simulink model "Monitor"  (R2022b)
settings: Solver=ode1  StartTime=0.0  StopTime=0.2  FixedStep=ctrlConst.TsSwitch  MaxStep=1e-6  RelTol=1e-3  EnableMultiTasking=on
PreLoadFcn:
  | %rtwdemo_pmsmfoc_data
StartFcn:
  | %clear executionProfile
StopFcn:
  | %try
  | %  AddExecutionProfileToDataInspector();
  | %end
undefined symbols (not defined in the file or in its folder): dataIphaOfsRawMon_C, facAdc2iPhMon_C, facAdc2uDclnkMon_C, KiRslvMonPI_C, KpRslvMonPI_C, Ld, Lq, Rss, SC_pMon_P, SC_PsiMon_P, tauTrqMonLv2_C, tauUdcPT1Mon_C, trqASCThdMonLv2_C, trqCmpThdMonLv2_C, Ts_10ms, Ts_1ms, Tsw
libraries: MathLib x14, IOLib x1, simulink x1
(part 1 of 2)
settings Model: Creator=The MathWorks, Inc.  LastModifiedBy=M00039784
settings SolverCC: AlgebraicLoopSolver=TrustRegion  InsertRTBMode=Never (minimum delay)
settings DataIOCC: LimitDataPoints=on  SaveFormat=Array  SaveOutput=off  SaveTime=off
settings OptimizationCC: DefaultParameterBehavior=Inlined  UseDivisionForNetSlopeComputation=on  UseFloatMulNetSlope=on  DefaultUnderspecifiedDataType=single  InlineInvariantSignals=on  PassReuseOutputArgsAs=Individual arguments  ExpressionDepthLimit=2147483647  ZeroExternalMemoryAtStartup=off  ZeroInternalMemoryAtStartup=off  NoFixptDivByZeroProtection=on  EfficientFloat2IntCast=on  LifeSpan=1  EfficientTunableParamExpr=on
settings DebuggingCC: ReadBeforeWriteMsg=DisableAll  WriteAfterWriteMsg=DisableAll  WriteAfterReadMsg=DisableAll  AlgebraicLoopMsg=none  MultiTaskDSMMsg=none  SingleTaskRateTransMsg=error  IntegerOverflowMsg=none  ParameterPrecisionLossMsg=none  FcnCallInpInsideContextMsg=warning  BusObjectLabelMismatch=none  AssertControl=DisableAll  AllowSymbolicDim=off  StateNameClashWarn=warning  SFUnexpectedBacktrackingDiag=warning  SFNoUnconditionalDefaultTransitionDiag=warning  SFExecutionAtInitializationDiag=none  SFMachineParentedDataDiag=warning  IntegerSaturationMsg=none  UnitsInconsistencyMsg=none  ArithmeticOperatorsInVariantConditions=warning
settings HardwareCC: ProdBitPerPointer=32  ProdBitPerSizeT=32  ProdBitPerPtrDiffT=32  ProdLargestAtomicFloat=None  ProdWordSize=32  ProdHWDeviceType=Infineon->TriCore
settings ModelReferenceCC: UpdateModelReferenceTargets=IfOutOfDate  EnableRefExpFcnMdlSchedulingChecks=on  ModelReferenceNumInstancesAllowed=Single  PropagateSignalLabelsOutOfModel=off
settings SFSimCC: SFSimEcho=off  SimUseLocalCustomCode=off  MATLABDynamicMemAlloc=off  CustomCodeUndefinedFunction=UseInterfaceOnly
settings RTWCC: Description=Embedded Coder  SystemTargetFile=ert.tlc  GenCodeOnly=on  GenerateMakefile=off  TemplateMakefile=ec_target.tmf  RTWVerbose=off  RTWUseLocalCustomCode=off  PortableWordSizes=on  CodeExecutionProfiling=on  CodeProfilingSaveOptions=AllData  CodeProfilingInstrumentation=detailed
settings CodeAppCC: ForceParamTrailComments=on  IgnoreCustomStorageClasses=off  IgnoreTestpoints=on  MaxIdLength=64  SimulinkDataObjDesc=on  MATLABFcnDesc=on  CustomSymbolStrGlobalVar=monitor_rt$N$M  CustomSymbolStrType=monitor_$N$M  CustomSymbolStrFcn=$N$M$F  CustomSymbolStrFcnArg=$I$N$M  CustomSymbolStrMacro=$N$M  InsertBlockDesc=on  StateflowObjectComments=on  MATLABSourceComments=on  InternalIdentifier=Classic
settings ERTTargetCC: UtilityFuncGeneration=Shared location  MultiwordLength=2048  CombineSignalStateStructs=on  SupportAbsoluteTime=off  SupportNonFinite=off  SupportComplex=off  SupportNonInlinedSFcns=on  RemoveResetFunc=off  ParenthesesLevel=Maximum  GenerateASAP2=on  InlinedParameterPlacement=NonHierarchical  ERTCustomFileTemplate=example_file_process.tlc  EnableDataOwnership=on  ConvertIfToSwitch=off  SuppressUnreachableDefaultCases=off  MemSecPackage=Simulink  MemSecDataConstants=MemConst  MemSecDataParameters=MemConstVolatile
settings ConfigComp: CovMetricSettings=dcmtrzow  CovHTMLOptions=-aTS=1 -bRG=1 -bTC=1 -hTR=0 -nFC=0 -scm=1 -bcm=1 -xEv=0  CovSaveCumulativeToWorkspaceVar=on  CovSaveSingleToWorkspaceVar=on  CovExternalEMLEnable=off  CovSFcnEnable=off
settings SimscapeCC: SimscapeNormalizeSystem=off

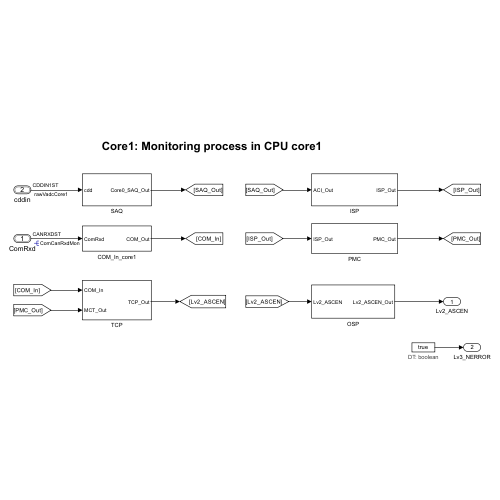
[thumbnail: Simulink's stored preview of the top-level diagram]
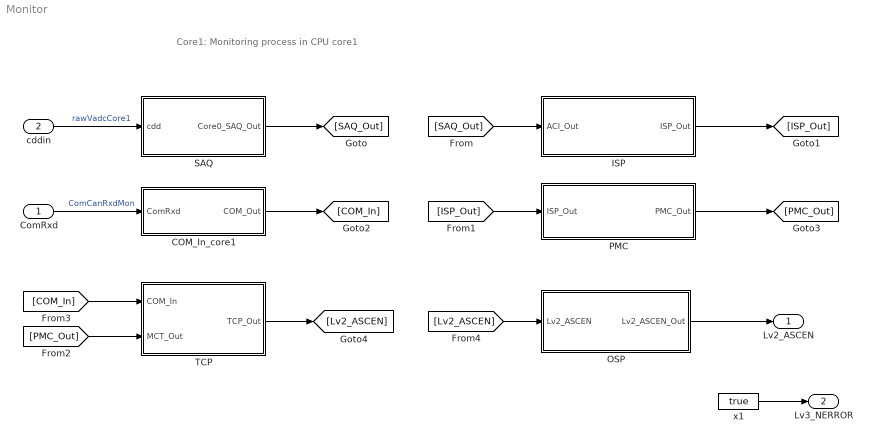
== system Monitor ==
  note: Core1: Monitoring process in CPU core1
  ComRxd : Inport  OutDataTypeStr=Bus: CANRXDST  SampleTime=Ts_10ms  BusOutputAsStruct=on
  cddin : Inport  Port=2  OutDataTypeStr=Bus: CDDIN1ST  SampleTime=Tsw  BusOutputAsStruct=on
  COM_In_core1 : Subsystem
  ISP : Subsystem
      settings: RTWSystemCode=Nonreusable function
  OSP : Subsystem
  PMC : Subsystem  SystemSampleTime=Tsw
  SAQ : Subsystem
  TCP : Subsystem  SystemSampleTime=Tsw
  x1 : Constant  Value=true  OutDataTypeStr=boolean
      settings: AttributesFormatString=DT: %<OutDataTypeStr>
  Lv2_ASCEN : Outport  VectorParamsAs1DForOutWhenUnconnected=off
  Lv3_NERROR : Outport  Port=2  VectorParamsAs1DForOutWhenUnconnected=off
  wires:
  SAQ/1(Core0_SAQ_Out) -> [SAQ_Out]
  cddin/1 -> SAQ/1(cdd)  "rawVadcCore1"
  [SAQ_Out] -> ISP/1(ACI_Out)
  ComRxd/1 -> COM_In_core1/1(ComRxd)  "ComCanRxdMon"
  COM_In_core1/1(COM_Out) -> [COM_In]
  ISP/1(ISP_Out) -> [ISP_Out]
  [ISP_Out] -> PMC/1(ISP_Out)
  PMC/1(PMC_Out) -> [PMC_Out]
  [PMC_Out] -> TCP/2(MCT_Out)
  [COM_In] -> TCP/1(COM_In)
  x1/1 -> Lv3_NERROR/1
  TCP/1(TCP_Out) -> [Lv2_ASCEN]
  [Lv2_ASCEN] -> OSP/1(Lv2_ASCEN)
  OSP/1(Lv2_ASCEN_Out) -> Lv2_ASCEN/1

== system Monitor/COM_In_core1 ==
  ComRxd : Inport  OutDataTypeStr=Bus: CANRXDST
  MSG04 : Subsystem
  Sel : BusSelector  OutputSignals=msg_MSG_04
  bus : BusCreator  Inputs=1
  COM_Out : Outport  VectorParamsAs1DForOutWhenUnconnected=off
  wires:
  ComRxd/1 -> Sel/1
  bus/1 -> COM_Out/1
  Sel/1 -> MSG04/1(MSG04)  "<msg_MSG_04>"
  MSG04/1(Com_MSG04) -> bus/1  "Com_Msg04"

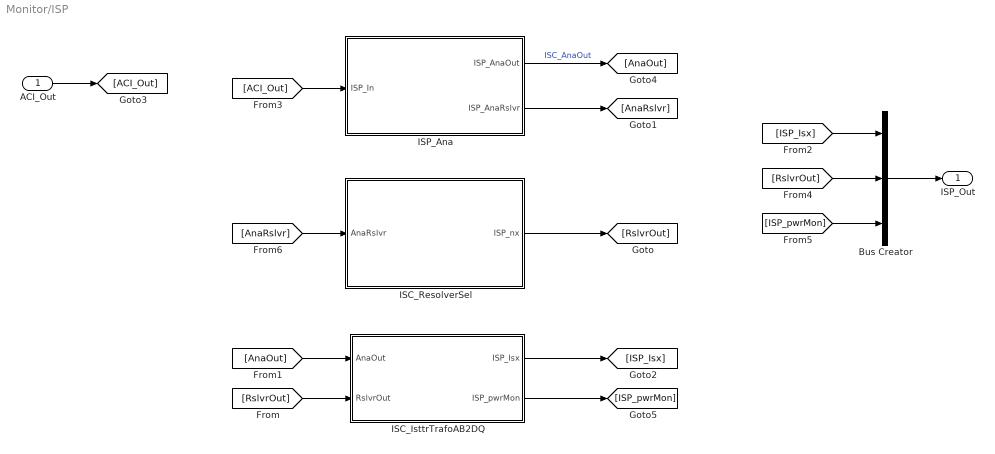
== system Monitor/ISP ==
  ACI_Out : Inport
  Bus Creator : BusCreator  Inputs=3
  ISC_IsttrTrafoAB2DQ : Subsystem
  ISC_ResolverSel : Subsystem
  ISP_Ana : Subsystem
  ISP_Out : Outport  VectorParamsAs1DForOutWhenUnconnected=off
  wires:
  ACI_Out/1 -> [ACI_Out]
  [ACI_Out] -> ISP_Ana/1(ISP_In)
  ISP_Ana/1(ISP_AnaOut) -> [AnaOut]  "ISC_AnaOut"
  [AnaOut] -> ISC_IsttrTrafoAB2DQ/1(AnaOut)
  ISP_Ana/2(ISP_AnaRslvr) -> [AnaRslvr]
  [RslvrOut] -> ISC_IsttrTrafoAB2DQ/2(RslvrOut)
  ISC_IsttrTrafoAB2DQ/1(ISP_Isx) -> [ISP_Isx]
  Bus Creator/1 -> ISP_Out/1
  [ISP_Isx] -> Bus Creator/1
  [RslvrOut] -> Bus Creator/2
  [AnaRslvr] -> ISC_ResolverSel/1(AnaRslvr)
  ISC_ResolverSel/1(ISP_nx) -> [RslvrOut]
  ISC_IsttrTrafoAB2DQ/2(ISP_pwrMon) -> [ISP_pwrMon]
  [ISP_pwrMon] -> Bus Creator/3

== system Monitor/OSP ==
  note: User is resposible to collect all the digital signals and resTolve to workspce
      | here the constant are only for reference
  Lv2_ASCEN : Inport
  SetDo7 : IOLib/SetDo  SystemSampleTime=-1
      link override Enumerated Constant: Value=EGPO.L2ASCEN
  Lv2_ASCEN_Out : Outport  VectorParamsAs1DForOutWhenUnconnected=off
  wires:
  Lv2_ASCEN/1 -> Lv2_ASCEN_Out/1

== system Monitor/PMC ==
  ISP_Out : Inport
  Bus Creator : BusCreator  Inputs=1
  Bus Selector1 : BusSelector  OutputSignals=ISP_Isx.ISP_isdMon,ISP_Isx.ISP_isqMon,ISP_nxMon.ISP_wElecMon
  PMC_PsmMdl : Subsystem
  PMC_TrqCal : Subsystem
  Terminator1 : Terminator
  Terminator2 : Terminator
  PMC_Out : Outport  VectorParamsAs1DForOutWhenUnconnected=off
  wires:
  ISP_Out/1 -> Bus Selector1/1
  Bus Selector1/1 -> PMC_PsmMdl/1(ISP_Isd)  "<ISP_isdMon>"
  Bus Selector1/2 -> PMC_PsmMdl/2(ISP_Isq)  "<ISP_isqMon>"
  Bus Selector1/3 -> PMC_PsmMdl/3(ISP_wElec)  "<ISP_wElecMon>"
  PMC_PsmMdl/1(PMC_IsdFlt1ms) -> PMC_TrqCal/1(PMC_IsdFlt1ms)
  PMC_PsmMdl/2(PMC_IsqFlt1ms) -> PMC_TrqCal/2(PMC_IsqFlt1ms)
  PMC_PsmMdl/3(PMC_PsiExc) -> PMC_TrqCal/3(PMC_psiExc)
  PMC_PsmMdl/4(PMC_LqSubLd) -> PMC_TrqCal/4(PMC_LqSubLd)
  PMC_PsmMdl/5(PMC_Ld) -> Terminator1/1
  PMC_PsmMdl/6(PMC_Rs) -> Terminator2/1
  Bus Creator/1 -> PMC_Out/1
  PMC_TrqCal/1(PMC_trqMon) -> Bus Creator/1

== system Monitor/SAQ ==
  cdd : Inport
  cddRt : Subsystem
  Core0_SAQ_Out : Outport  VectorParamsAs1DForOutWhenUnconnected=off
      settings: AttributesFormatString=Disable Action: %<OutputWhenDisabled>
  wires:
  cdd/1 -> cddRt/1(cddSt)
  cddRt/1(cddSig) -> Core0_SAQ_Out/1  "cddRt"

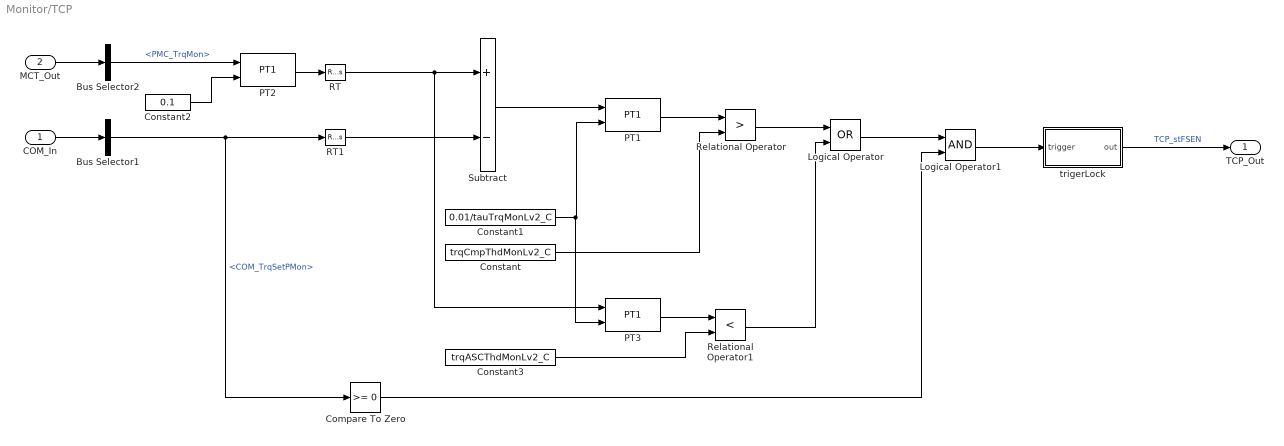
== system Monitor/TCP ==
  COM_In : Inport
  MCT_Out : Inport  Port=2
  Bus Selector1 : BusSelector  OutputSignals=Com_Msg04.COM_TrqSetPMon
  Bus Selector2 : BusSelector  OutputSignals=PMC_TrqMon
  Compare To Zero : simulink/Logic and Bit Operations/Compare To Zero  relop=>=  OutDataTypeStr=boolean
  Constant : Constant  Value=trqCmpThdMonLv2_C
  Constant1 : Constant  Value=0.01/tauTrqMonLv2_C
  Constant2 : Constant  Value=0.1
  Constant3 : Constant  Value=trqASCThdMonLv2_C
  Logical Operator : Logic  Operator=OR  AllPortsSameDT=off  OutDataTypeStr=boolean
  Logical Operator1 : Logic  AllPortsSameDT=off  OutDataTypeStr=boolean
  PT1 : MathLib/PT1
  PT2 : MathLib/PT1
  PT3 : MathLib/PT1
  RT : RateTransition  OutPortSampleTime=Ts_10ms
  RT1 : RateTransition  OutPortSampleTime=Ts_10ms
  Relational Operator : RelationalOperator  Operator=>  OutDataTypeStr=boolean  RndMeth=Simplest  InputSameDT=off
  Relational Operator1 : RelationalOperator  Operator=<  OutDataTypeStr=boolean  RndMeth=Simplest  InputSameDT=off
  Subtract : Sum  Inputs=+-
  trigerLock : MATLAB Function
  TCP_Out : Outport  VectorParamsAs1DForOutWhenUnconnected=off
  wires:
  COM_In/1 -> Bus Selector1/1
  MCT_Out/1 -> Bus Selector2/1
  Bus Selector1/1 -> Compare To Zero/1, RT1/1  "<COM_TrqSetPMon>"
  PT1/1 -> Relational Operator/1
  Constant/1 -> Relational Operator/2
  Logical Operator1/1 -> trigerLock/1(trigger)
  Subtract/1 -> PT1/1
  Constant1/1 -> PT3/2, PT1/2
  Constant2/1 -> PT2/2
  Bus Selector2/1 -> PT2/1  "<PMC_TrqMon>"
  PT2/1 -> RT/1
  RT/1 -> PT3/1, Subtract/1
  RT1/1 -> Subtract/2
  Constant3/1 -> Relational Operator1/2
  Relational Operator1/1 -> Logical Operator/2
  Logical Operator/1 -> Logical Operator1/1
  Compare To Zero/1 -> Logical Operator1/2
  trigerLock/1(out) -> TCP_Out/1  "TCP_stFSEN"
  Relational Operator/1 -> Logical Operator/1
  PT3/1 -> Relational Operator1/1

== system Monitor/COM_In_core1/MSG04 ==
  MSG04 : Inport
  Data Type Conversion : DataTypeConversion  OutDataTypeStr=Enum: ECM  SaturateOnIntegerOverflow=off  RndMeth=Floor
  Data Type Conversion1 : DataTypeConversion  OutDataTypeStr=uint16  SaturateOnIntegerOverflow=off  RndMeth=Floor
  RT{,1..3} (4 alike) : RateTransition
  Sel : BusSelector  OutputSignals=MSG04_NSetP,MSG04_TrqSetP,MSG04_UdcSetP,MSG04_stModeReq
  bus : BusCreator  Inputs=4
  Com_MSG04 : Outport  VectorParamsAs1DForOutWhenUnconnected=off
  wires:
  MSG04/1 -> Sel/1
  bus/1 -> Com_MSG04/1
  RT/1 -> bus/1  "COM_NSetPMon"
  Sel/1 -> RT/1  "<MSG04_NSetP>"
  RT1/1 -> bus/2  "COM_TrqSetPMon"
  Sel/2 -> RT1/1  "<MSG04_TrqSetP>"
  RT2/1 -> bus/3  "COM_UdcSetPMon"
  Sel/3 -> RT2/1  "<MSG04_UdcSetP>"
  RT3/1 -> bus/4  "COM_stModeReqMon"
  Sel/4 -> Data Type Conversion1/1  "<MSG04_stModeReq>"
  Data Type Conversion/1 -> RT3/1
  Data Type Conversion1/1 -> Data Type Conversion/1

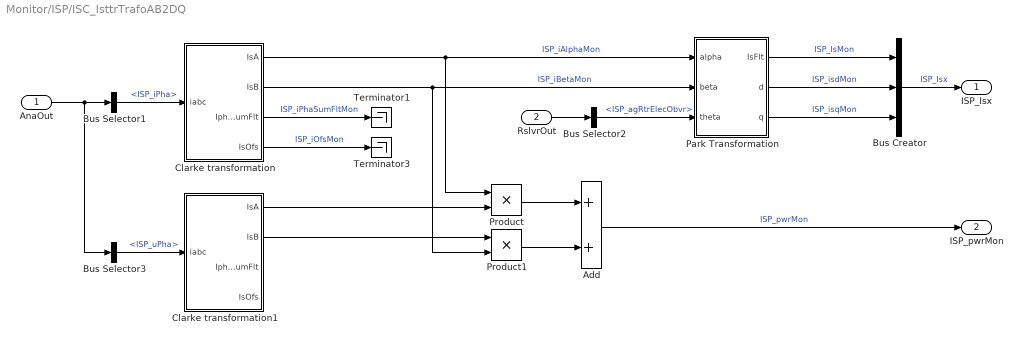
== system Monitor/ISP/ISC_IsttrTrafoAB2DQ ==
  AnaOut : Inport
  RslvrOut : Inport  Port=2
  Add : Sum
  Bus Creator : BusCreator  Inputs=3
  Bus Selector1 : BusSelector  OutputSignals=ISP_iPha
  Bus Selector2 : BusSelector  OutputSignals=ISP_agRtrElecObvr
  Bus Selector3 : BusSelector  OutputSignals=ISP_uPha
  Clarke transformation : Subsystem
  Clarke transformation1 : Subsystem
  Park Transformation : Subsystem
  Product : Product
  Product1 : Product
  Terminator1 : Terminator
  Terminator3 : Terminator
  ISP_Isx : Outport  VectorParamsAs1DForOutWhenUnconnected=off
  ISP_pwrMon : Outport  Port=2  VectorParamsAs1DForOutWhenUnconnected=off
  wires:
  Bus Creator/1 -> ISP_Isx/1  "ISP_Isx"
  Clarke transformation/4(IsOfs) -> Terminator3/1  "ISP_iOfsMon"
  AnaOut/1 -> Bus Selector3/1, Bus Selector1/1
  Park Transformation/2(d) -> Bus Creator/2  "ISP_isdMon"
  Park Transformation/3(q) -> Bus Creator/3  "ISP_isqMon"
  Clarke transformation/1(IsA) -> Product/1, Park Transformation/1(alpha)  "ISP_iAlphaMon"
  Clarke transformation/2(IsB) -> Product1/2, Park Transformation/2(beta)  "ISP_iBetaMon"
  Park Transformation/1(IsFlt) -> Bus Creator/1  "ISP_IsMon"
  Bus Selector1/1 -> Clarke transformation/1(iabc)  "<ISP_iPha>"
  Clarke transformation/3(IphaSumFlt) -> Terminator1/1  "ISP_iPhaSumFltMon"
  RslvrOut/1 -> Bus Selector2/1
  Bus Selector2/1 -> Park Transformation/3(theta)  "<ISP_agRtrElecObvr>"
  Bus Selector3/1 -> Clarke transformation1/1(iabc)  "<ISP_uPha>"
  Clarke transformation1/1(IsA) -> Product/2
  Clarke transformation1/2(IsB) -> Product1/1
  Product/1 -> Add/1
  Product1/1 -> Add/2
  Add/1 -> ISP_pwrMon/1  "ISP_pwrMon"

== system Monitor/ISP/ISC_ResolverSel ==
  note: Theta Selection
  note: if the resolver flag ture, the output angle and electric frequency are equal to the observer
      | if the resolver flag false, the output andle and electric frequency are equal to the dirct atan2 calculation.
  AnaRslvr : Inport
  Bus Creator : BusCreator  Inputs=4
  Bus Selector6 : BusSelector  OutputSignals=ISP_agRtrElecObvr,ISP_frqElecObvr
  Divide : Product  Inputs=*/
  NpMotorDivNpResolver1 : Constant  Value=SC_pMon_P  OutDataTypeStr=Inherit: Inherit via back propagation
  Saturation : Saturate  UpperLimit=18000  LowerLimit=-18000
  fac2piFrq2w : Gain  Gain=2*pi  SaturateOnIntegerOverflow=on  OutDataTypeStr=Inherit: Same as input  ParamDataTypeStr=Inherit: Same as input
  facf2n : Gain  Gain=60  SaturateOnIntegerOverflow=on  OutDataTypeStr=Inherit: Same as input  ParamDataTypeStr=Inherit: Same as input
  ISP_nx : Outport  VectorParamsAs1DForOutWhenUnconnected=off
  wires:
  AnaRslvr/1 -> Bus Selector6/1
  Bus Creator/1 -> ISP_nx/1  "ISP_nxMon"
  facf2n/1 -> Divide/1
  fac2piFrq2w/1 -> Bus Creator/3  "ISP_wElecMon"
  Bus Selector6/1 -> Bus Creator/1  "<ISP_agRtrElecObvr>"
  Bus Selector6/2 -> facf2n/1, fac2piFrq2w/1, Bus Creator/2  "<ISP_frqElecObvr>"
  Saturation/1 -> Bus Creator/4  "ISP_nMon"
  Divide/1 -> Saturation/1
  NpMotorDivNpResolver1/1 -> Divide/2

== system Monitor/ISP/ISP_Ana ==
  note: Input Signal Calculation (Analogue)
  ISP_In : Inport
  Bus Creator : BusCreator  Inputs=3
  Bus Creator1 : BusCreator  Inputs=5
  Bus Selector1 : BusSelector  OutputSignals=SAQ_SINH,SAQ_SINL,SAQ_COSH,SAQ_COSL
  Bus Selector2 : BusSelector  OutputSignals=SAQ_HVUEX
  Bus Selector3 : BusSelector  OutputSignals=SAQ_IPH1B,SAQ_IPH2B,SAQ_IPH3B  OutputAsBus=on
  Bus Selector4 : BusSelector  OutputSignals=SAQ_DUTY1,SAQ_DUTY2,SAQ_DUTY3  OutputAsBus=on
  ISP_AnaCalnIpha : Subsystem
  ISP_AnaCalnPosCalnMon : Subsystem  SystemSampleTime=Tsw
      settings: RTWSystemCode=Nonreusable function
  ISP_AnaCalnUdcLnk : Subsystem  SystemSampleTime=Tsw
  ISP_AnaCalnUpha : Subsystem
  tiPerd : Constant  Value=100  OutDataTypeStr=single
  ISP_AnaOut : Outport  VectorParamsAs1DForOutWhenUnconnected=off
  ISP_AnaRslvr : Outport  Port=2  VectorParamsAs1DForOutWhenUnconnected=off
  wires:
  ISP_In/1 -> Bus Selector3/1, Bus Selector4/1, Bus Selector1/1, Bus Selector2/1
  ISP_AnaCalnIpha/1(ISP_iPha) -> Bus Creator/2  "ISP_iPha"
  ISP_AnaCalnUdcLnk/1(ISP_uDcFltMon) -> Bus Creator/3
  Bus Creator/1 -> ISP_AnaOut/1
  Bus Selector1/1 -> ISP_AnaCalnPosCalnMon/1(sinH)  "<SAQ_SINH>"
  Bus Selector1/2 -> ISP_AnaCalnPosCalnMon/2(sinL)  "<SAQ_SINL>"
  Bus Selector1/3 -> ISP_AnaCalnPosCalnMon/3(cosH)  "<SAQ_COSH>"
  Bus Selector1/4 -> ISP_AnaCalnPosCalnMon/4(cosL)  "<SAQ_COSL>"
  tiPerd/1 -> ISP_AnaCalnPosCalnMon/5(tiPerd)
  ISP_AnaCalnPosCalnMon/3(ISP_frqElecObvr) -> Bus Creator1/3
  ISP_AnaCalnPosCalnMon/2(ISP_agRtrElecObvr) -> Bus Creator1/2
  ISP_AnaCalnPosCalnMon/4(ISP_agRtrElecAtan2) -> Bus Creator1/4
  ISP_AnaCalnPosCalnMon/1(dAngle) -> Bus Creator1/1
  ISP_AnaCalnPosCalnMon/5(ISP_frqElecCaln) -> Bus Creator1/5
  Bus Creator1/1 -> ISP_AnaRslvr/1  "ISP_RslvrOut"
  ISP_AnaCalnUpha/1(ISP_uPha) -> Bus Creator/1  "ISP_uPha"
  Bus Selector2/1 -> ISP_AnaCalnUdcLnk/1(CddHvMcu_dataDclnkRaw)  "<SAQ_HVUEX>"
  Bus Selector3/1 -> ISP_AnaCalnIpha/1(dataIPha)
  Bus Selector4/1 -> ISP_AnaCalnUpha/1(dataUPha)

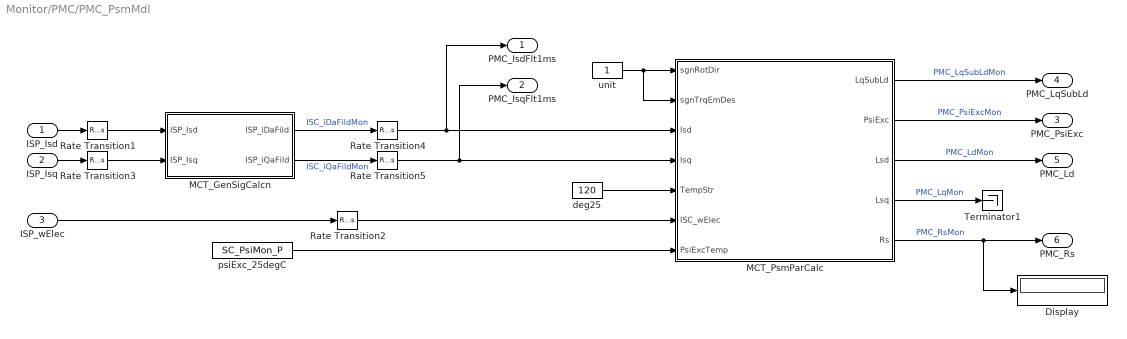
== system Monitor/PMC/PMC_PsmMdl ==
  ISP_Isd : Inport
  ISP_Isq : Inport  Port=2
  ISP_wElec : Inport  Port=3
  Display : Display
  MCT_GenSigCalcn : Subsystem
  MCT_PsmParCalc : Subsystem  TreatAsAtomicUnit=on  SystemSampleTime=Ts_1ms
  Rate Transition1 : RateTransition  OutPortSampleTime=Tsw
  Rate Transition2 : RateTransition  OutPortSampleTime=Ts_1ms
  Rate Transition3 : RateTransition  OutPortSampleTime=Tsw
  Rate Transition4 : RateTransition  OutPortSampleTime=Ts_1ms
  Rate Transition5 : RateTransition  OutPortSampleTime=Ts_1ms
  Terminator1 : Terminator
  deg25 : Constant  Value=120  OutDataTypeStr=single  SampleTime=Ts_1ms
  psiExc_25degC : Constant  Value=SC_PsiMon_P  OutDataTypeStr=single  SampleTime=Ts_1ms
  unit : Constant  OutDataTypeStr=uint8  SampleTime=Ts_1ms
  PMC_IsdFlt1ms : Outport  VectorParamsAs1DForOutWhenUnconnected=off
  PMC_IsqFlt1ms : Outport  Port=2  VectorParamsAs1DForOutWhenUnconnected=off
  PMC_PsiExc : Outport  Port=3  VectorParamsAs1DForOutWhenUnconnected=off
  PMC_LqSubLd : Outport  Port=4  VectorParamsAs1DForOutWhenUnconnected=off
  PMC_Ld : Outport  Port=5  VectorParamsAs1DForOutWhenUnconnected=off
  PMC_Rs : Outport  Port=6  VectorParamsAs1DForOutWhenUnconnected=off
  wires:
  MCT_PsmParCalc/5(Rs) -> Display/1, PMC_Rs/1  "PMC_RsMon"
  MCT_PsmParCalc/1(LqSubLd) -> PMC_LqSubLd/1  "PMC_LqSubLdMon"
  MCT_PsmParCalc/2(PsiExc) -> PMC_PsiExc/1  "PMC_PsiExcMon"
  Rate Transition5/1 -> PMC_IsqFlt1ms/1, MCT_PsmParCalc/4(Isq)
  Rate Transition3/1 -> MCT_GenSigCalcn/2(ISP_Isq)
  Rate Transition1/1 -> MCT_GenSigCalcn/1(ISP_Isd)
  MCT_GenSigCalcn/1(ISP_iDaFild) -> Rate Transition4/1  "ISC_iDaFildMon"
  ISP_Isq/1 -> Rate Transition3/1
  ISP_Isd/1 -> Rate Transition1/1
  MCT_GenSigCalcn/2(ISP_iQaFild) -> Rate Transition5/1  "ISC_iQaFildMon"
  MCT_PsmParCalc/3(Lsd) -> PMC_Ld/1  "PMC_LdMon"
  MCT_PsmParCalc/4(Lsq) -> Terminator1/1  "PMC_LqMon"
  deg25/1 -> MCT_PsmParCalc/5(TempStr)
  unit/1 -> MCT_PsmParCalc/2(sgnTrqEmDes), MCT_PsmParCalc/1(sgnRotDir)
  ISP_wElec/1 -> Rate Transition2/1
  Rate Transition2/1 -> MCT_PsmParCalc/6(ISC_wElec)
  psiExc_25degC/1 -> MCT_PsmParCalc/7(PsiExcTemp)
  Rate Transition4/1 -> PMC_IsdFlt1ms/1, MCT_PsmParCalc/3(Isd)

== system Monitor/PMC/PMC_TrqCal ==
  PMC_IsdFlt1ms : Inport
  PMC_IsqFlt1ms : Inport  Port=2
  PMC_psiExc : Inport  Port=3
  PMC_LqSubLd : Inport  Port=4
  Add : Sum  Inputs=+-
  Constant : Constant  Value=SC_pMon_P
  Constant1 : Constant  Value=3  OutDataTypeStr=single
  Product : Product
  Product1 : Product
  Product2 : Product  Inputs=3
  Product3 : Product
  PMC_trqMon : Outport  VectorParamsAs1DForOutWhenUnconnected=off
  wires:
  Product3/1 -> PMC_trqMon/1  "PMC_TrqMon"
  PMC_IsdFlt1ms/1 -> Product2/2
  PMC_IsqFlt1ms/1 -> Product2/1, Product1/2
  Constant1/1 -> Product/1
  Constant/1 -> Product/2
  PMC_psiExc/1 -> Product1/1
  PMC_LqSubLd/1 -> Product2/3
  Product1/1 -> Add/1
  Product2/1 -> Add/2
  Product/1 -> Product3/1
  Add/1 -> Product3/2

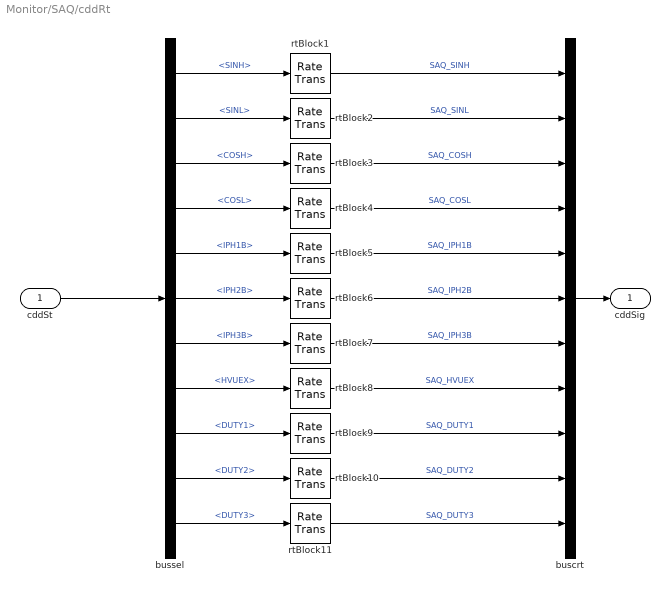
== system Monitor/SAQ/cddRt ==
  cddSt : Inport
  buscrt : BusCreator  Inputs=11
  bussel : BusSelector  OutputSignals=SINH,SINL,COSH,COSL,IPH1B,IPH2B,IPH3B,HVUEX,DUTY1,DUTY2,DUTY3
  rtBlock{1..11} (11 alike) : RateTransition  OutPortSampleTimeOpt=Inherit
  cddSig : Outport
  wires:
  cddSt/1 -> bussel/1
  buscrt/1 -> cddSig/1
  bussel/1 -> rtBlock1/1  "<SINH>"
  rtBlock1/1 -> buscrt/1  "SAQ_SINH"
  bussel/2 -> rtBlock2/1  "<SINL>"
  rtBlock2/1 -> buscrt/2  "SAQ_SINL"
  bussel/3 -> rtBlock3/1  "<COSH>"
  rtBlock3/1 -> buscrt/3  "SAQ_COSH"
  bussel/4 -> rtBlock4/1  "<COSL>"
  rtBlock4/1 -> buscrt/4  "SAQ_COSL"
  bussel/5 -> rtBlock5/1  "<IPH1B>"
  rtBlock5/1 -> buscrt/5  "SAQ_IPH1B"
  bussel/6 -> rtBlock6/1  "<IPH2B>"
  rtBlock6/1 -> buscrt/6  "SAQ_IPH2B"
  bussel/7 -> rtBlock7/1  "<IPH3B>"
  rtBlock7/1 -> buscrt/7  "SAQ_IPH3B"
  bussel/8 -> rtBlock8/1  "<HVUEX>"
  rtBlock8/1 -> buscrt/8  "SAQ_HVUEX"
  bussel/9 -> rtBlock9/1  "<DUTY1>"
  rtBlock9/1 -> buscrt/9  "SAQ_DUTY1"
  bussel/10 -> rtBlock10/1  "<DUTY2>"
  rtBlock10/1 -> buscrt/10  "SAQ_DUTY2"
  bussel/11 -> rtBlock11/1  "<DUTY3>"
  rtBlock11/1 -> buscrt/11  "SAQ_DUTY3"

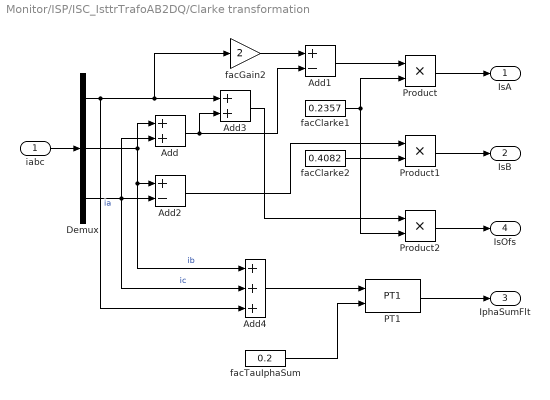
== system Monitor/ISP/ISC_IsttrTrafoAB2DQ/Clarke transformation ==
  iabc : Inport
  Add : Sum
  Add1 : Sum  Inputs=+-
  Add2 : Sum  Inputs=+-
  Add3 : Sum
  Add4 : Sum  Inputs=+++
  Demux : Demux  Outputs=3
  PT1 : MathLib/PT1
  Product : Product
  Product1 : Product  OutDataTypeStr=single
  Product2 : Product  OutDataTypeStr=single
  facClarke1 : Constant  Value=0.2357  OutDataTypeStr=single
  facClarke2 : Constant  Value=0.4082  OutDataTypeStr=single
  facGain2 : Gain  Gain=2
  facTauIphaSum : Constant  Value=0.2  OutDataTypeStr=single
  IsA : Outport  VectorParamsAs1DForOutWhenUnconnected=off
  IsB : Outport  Port=2  VectorParamsAs1DForOutWhenUnconnected=off
  IphaSumFlt : Outport  Port=3  VectorParamsAs1DForOutWhenUnconnected=off
  IsOfs : Outport  Port=4  VectorParamsAs1DForOutWhenUnconnected=off
  wires:
  Demux/1 -> Add4/3, Add3/1, facGain2/1  "ia"
  iabc/1 -> Demux/1
  Demux/3 -> Add4/2, Add2/2, Add/2  "ic"
  Demux/2 -> Add4/1, Add2/1, Add/1  "ib"
  facGain2/1 -> Add1/1
  Add/1 -> Add1/2, Add3/2
  Add1/1 -> Product/1
  Product/1 -> IsA/1
  facClarke1/1 -> Product2/2, Product/2
  Add2/1 -> Product1/1
  facClarke2/1 -> Product1/2
  Product1/1 -> IsB/1
  Add3/1 -> Product2/1
  Product2/1 -> IsOfs/1
  PT1/1 -> IphaSumFlt/1
  facTauIphaSum/1 -> PT1/2
  Add4/1 -> PT1/1

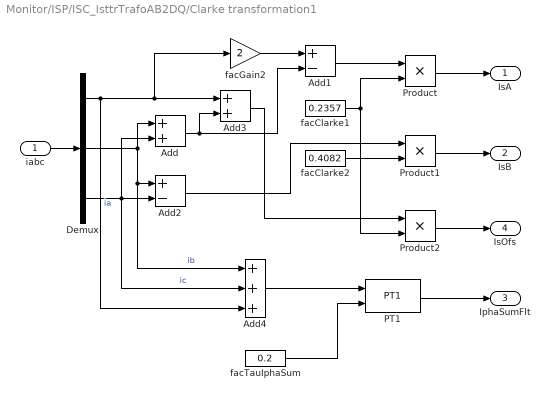
== system Monitor/ISP/ISC_IsttrTrafoAB2DQ/Clarke transformation1 ==
  iabc : Inport
  Add : Sum
  Add1 : Sum  Inputs=+-
  Add2 : Sum  Inputs=+-
  Add3 : Sum
  Add4 : Sum  Inputs=+++
  Demux : Demux  Outputs=3
  PT1 : MathLib/PT1  SystemSampleTime=-1  VariantActivationTime=update diagram  Latency=0  AutoFrameSizeCalculation=off
  Product : Product
  Product1 : Product  OutDataTypeStr=single
  Product2 : Product  OutDataTypeStr=single
  facClarke1 : Constant  Value=0.2357  OutDataTypeStr=single
  facClarke2 : Constant  Value=0.4082  OutDataTypeStr=single
  facGain2 : Gain  Gain=2
  facTauIphaSum : Constant  Value=0.2  OutDataTypeStr=single
  IsA : Outport  VectorParamsAs1DForOutWhenUnconnected=off
  IsB : Outport  Port=2  VectorParamsAs1DForOutWhenUnconnected=off
  IphaSumFlt : Outport  Port=3  VectorParamsAs1DForOutWhenUnconnected=off
  IsOfs : Outport  Port=4  VectorParamsAs1DForOutWhenUnconnected=off
  wires:
  Add4/1 -> PT1/1
  facTauIphaSum/1 -> PT1/2
  PT1/1 -> IphaSumFlt/1
  Product2/1 -> IsOfs/1
  Add3/1 -> Product2/1
  Product1/1 -> IsB/1
  facClarke2/1 -> Product1/2
  Add2/1 -> Product1/1
  facClarke1/1 -> Product/2, Product2/2
  Product/1 -> IsA/1
  Add1/1 -> Product/1
  Add/1 -> Add3/2, Add1/2
  facGain2/1 -> Add1/1
  Demux/2 -> Add/1, Add2/1, Add4/1  "ib"
  Demux/3 -> Add/2, Add2/2, Add4/2  "ic"
  iabc/1 -> Demux/1
  Demux/1 -> facGain2/1, Add3/1, Add4/3  "ia"

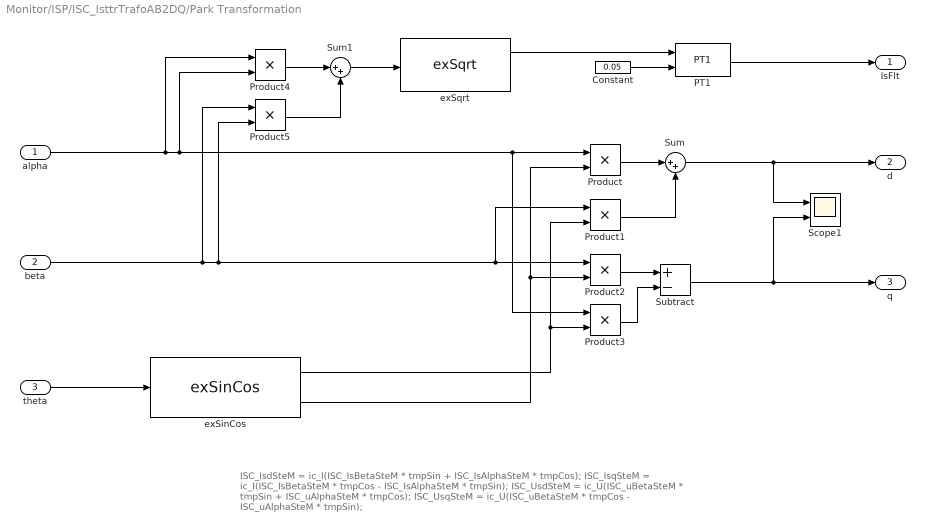
== system Monitor/ISP/ISC_IsttrTrafoAB2DQ/Park Transformation ==
  note: ISC_IsdSteM = ic_I(ISC_IsBetaSteM * tmpSin + ISC_IsAlphaSteM * tmpCos);
      | 			ISC_IsqSteM = ic_I(ISC_IsBetaSteM * tmpCos - ISC_IsAlphaSteM * tmpSin);
      |
      | 			ISC_UsdSteM = ic_U(ISC_uBetaSteM * tmpSin + ISC_uAlphaSteM * tmpCos);
      | 			ISC_UsqSteM = ic_U(ISC_uBetaSteM * tmpCos - ISC_uAlphaSteM * tmpSin);
  alpha : Inport
  beta : Inport  Port=2
  theta : Inport  Port=3
  Constant : Constant  Value=0.05  OutDataTypeStr=single
  PT1 : MathLib/PT1
  Product{,1..3,5} (5 alike) : Product  Priority=15  RndMeth=Zero
  Product4 : Product  Priority=15  OutDataTypeStr=Inherit: Inherit via back propagation  RndMeth=Zero
  Scope1 : Scope  NumInputPorts=2
  Subtract : Sum  Priority=40  Inputs=+-
  Sum : Sum  Priority=25  Inputs=|++
  Sum1 : Sum  Priority=25  Inputs=|++
  exSinCos : MathLib/exSinCos
  exSqrt : MathLib/exSqrt
  IsFlt : Outport  VectorParamsAs1DForOutWhenUnconnected=off
  d : Outport  Port=2  VectorParamsAs1DForOutWhenUnconnected=off
  q : Outport  Port=3  VectorParamsAs1DForOutWhenUnconnected=off
  wires:
  Subtract/1 -> q/1, Scope1/2
  Product3/1 -> Subtract/2
  Product2/1 -> Subtract/1
  Sum/1 -> Scope1/1, d/1
  Product1/1 -> Sum/2
  Product/1 -> Sum/1
  beta/1 -> Product5/1, Product5/2, Product2/1, Product1/1
  alpha/1 -> Product4/1, Product3/1, Product/1, Product4/2
  Product4/1 -> Sum1/1
  Product5/1 -> Sum1/2
  Sum1/1 -> exSqrt/1
  exSinCos/2 -> Product2/2, Product/2
  exSinCos/1 -> Product3/2, Product1/2
  theta/1 -> exSinCos/1
  PT1/1 -> IsFlt/1
  exSqrt/1 -> PT1/1
  Constant/1 -> PT1/2

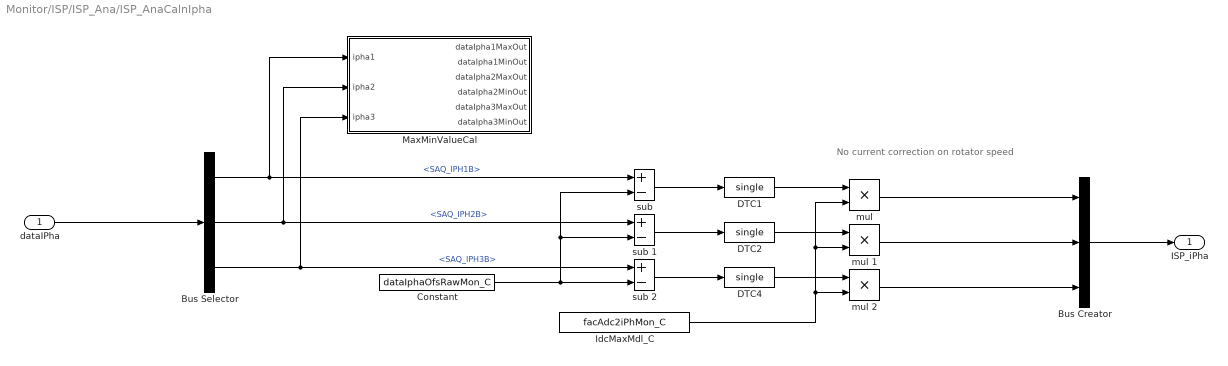
== system Monitor/ISP/ISP_Ana/ISP_AnaCalnIpha ==
  note: No current correction on rotator speed
  dataIPha : Inport
  Bus Creator : BusCreator  Inputs=3
  Bus Selector : BusSelector  OutputSignals=SAQ_IPH1B,SAQ_IPH2B,SAQ_IPH3B
  Constant : Constant  Value=dataIphaOfsRawMon_C  OutDataTypeStr=uint16
  DTC1 : DataTypeConversion  OutDataTypeStr=single  SaturateOnIntegerOverflow=off  RndMeth=Floor
  DTC2 : DataTypeConversion  OutDataTypeStr=single  SaturateOnIntegerOverflow=off  RndMeth=Floor
  DTC4 : DataTypeConversion  OutDataTypeStr=single  SaturateOnIntegerOverflow=off  RndMeth=Floor
  IdcMaxMdl_C : Constant  Value=facAdc2iPhMon_C
      mask Display:
      | tmpx = get_param(gcbh,'Value');
      | a= evalin('base',[tmpx,'.Value;']);
      | disp([tmpx,': ',num2str(a)]);
  MaxMinValueCal : MATLAB Function  TreatAsAtomicUnit=on  SystemSampleTime=Tsw
  mul : Product  OutDataTypeStr=single
  mul 1 : Product  OutDataTypeStr=single
  mul 2 : Product  OutDataTypeStr=single
  sub : Sum  Inputs=+-  OutDataTypeStr=single
  sub 1 : Sum  Inputs=+-  OutDataTypeStr=single
  sub 2 : Sum  Inputs=+-  OutDataTypeStr=single
  ISP_iPha : Outport  VectorParamsAs1DForOutWhenUnconnected=off
  wires:
  DTC4/1 -> mul 2/1
  DTC2/1 -> mul 1/1
  DTC1/1 -> mul/1
  Constant/1 -> sub 2/2, sub 1/2, sub/2
  Bus Creator/1 -> ISP_iPha/1
  sub/1 -> DTC1/1
  IdcMaxMdl_C/1 -> mul/2, mul 1/2, mul 2/2
  sub 1/1 -> DTC2/1
  sub 2/1 -> DTC4/1
  Bus Selector/1 -> MaxMinValueCal/1(ipha1), sub/1  "<SAQ_IPH1B>"
  Bus Selector/2 -> sub 1/1, MaxMinValueCal/2(ipha2)  "<SAQ_IPH2B>"
  Bus Selector/3 -> sub 2/1, MaxMinValueCal/3(ipha3)  "<SAQ_IPH3B>"
  dataIPha/1 -> Bus Selector/1
  mul/1 -> Bus Creator/1
  mul 1/1 -> Bus Creator/2
  mul 2/1 -> Bus Creator/3

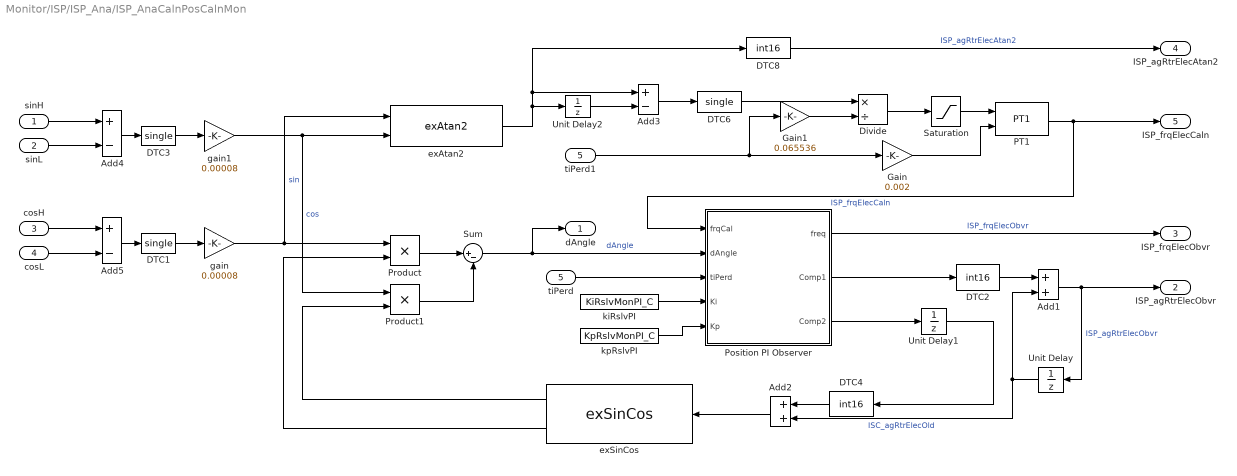
== system Monitor/ISP/ISP_Ana/ISP_AnaCalnPosCalnMon ==
  sinH : Inport
  sinL : Inport  Port=2
  cosH : Inport  Port=3
  cosL : Inport  Port=4
  tiPerd : Inport  Port=5
  Add1 : Sum  OutDataTypeStr=int16
  Add2 : Sum  OutDataTypeStr=uint16
  Add3 : Sum  Inputs=+-  OutDataTypeStr=int16
  Add4 : Sum  Inputs=+-  OutDataTypeStr=int16
  Add5 : Sum  Inputs=+-  OutDataTypeStr=int16
  DTC1 : DataTypeConversion  OutDataTypeStr=single  SaturateOnIntegerOverflow=off  RndMeth=Floor
  DTC2 : DataTypeConversion  OutDataTypeStr=int16  ConvertRealWorld=Stored Integer (SI)  RndMeth=Floor
  DTC3 : DataTypeConversion  OutDataTypeStr=single  SaturateOnIntegerOverflow=off  RndMeth=Floor
  DTC4 : DataTypeConversion  OutDataTypeStr=int16  ConvertRealWorld=Stored Integer (SI)  RndMeth=Floor
  DTC6 : DataTypeConversion  OutDataTypeStr=single  SaturateOnIntegerOverflow=off  RndMeth=Floor
  DTC8 : DataTypeConversion  OutDataTypeStr=int16  SaturateOnIntegerOverflow=off  RndMeth=Floor
  Divide : Product  Inputs=*/
  Gain : Gain  Gain=0.002
  Gain1 : Gain  Gain=0.065536
  PT1 : MathLib/PT1
  Position PI Observer : MATLAB Function  TreatAsAtomicUnit=on  SystemSampleTime=Tsw
  Product : Product
  Product1 : Product
  Saturation : Saturate  UpperLimit=2000  LowerLimit=-2000
  Sum : Sum  Inputs=|+-  SaturateOnIntegerOverflow=on
  Unit Delay : UnitDelay  SampleTime=-1  HasFrameUpgradeWarning=on
  Unit Delay1 : UnitDelay  SampleTime=-1  HasFrameUpgradeWarning=on
  Unit Delay2 : UnitDelay  SampleTime=-1  HasFrameUpgradeWarning=on
  exAtan2 : MathLib/exAtan2
  exSinCos : MathLib/exSinCos
  gain : Gain  Gain=0.00008  SaturateOnIntegerOverflow=on  OutDataTypeStr=Inherit: Same as input  ParamDataTypeStr=Inherit: Same as input
  gain1 : Gain  Gain=0.00008  SaturateOnIntegerOverflow=on  OutDataTypeStr=Inherit: Same as input  ParamDataTypeStr=Inherit: Same as input
  kiRslvPI : Constant  Value=KiRslvMonPI_C  OutDataTypeStr=single
  kpRslvPI : Constant  Value=KpRslvMonPI_C  OutDataTypeStr=single
  tiPerd1 : InportShadow  Port=5
  dAngle : Outport  VectorParamsAs1DForOutWhenUnconnected=off
  ISP_agRtrElecObvr : Outport  Port=2  VectorParamsAs1DForOutWhenUnconnected=off
  ISP_frqElecObvr : Outport  Port=3  VectorParamsAs1DForOutWhenUnconnected=off
  ISP_agRtrElecAtan2 : Outport  Port=4  VectorParamsAs1DForOutWhenUnconnected=off
  ISP_frqElecCaln : Outport  Port=5  VectorParamsAs1DForOutWhenUnconnected=off
  wires:
  exSinCos/1 -> Product1/2
  exSinCos/2 -> Product/2
  DTC1/1 -> gain/1
  DTC3/1 -> gain1/1
  Position PI Observer/1(freq) -> ISP_frqElecObvr/1  "ISP_frqElecObvr"
  Position PI Observer/2(Comp1) -> DTC2/1
  Add1/1 -> Unit Delay/1, ISP_agRtrElecObvr/1  "ISP_agRtrElecObvr"
  Add2/1 -> exSinCos/1
  Product/1 -> Sum/1
  Product1/1 -> Sum/2
  Sum/1 -> Position PI Observer/2(dAngle), dAngle/1  "dAngle"
  Unit Delay/1 -> Add2/2, Add1/2  "ISC_agRtrElecOld"
  Position PI Observer/3(Comp2) -> Unit Delay1/1
  gain/1 -> Product/1, exAtan2/1  "sin"
  gain1/1 -> exAtan2/2, Product1/1  "cos"
  tiPerd/1 -> Position PI Observer/3(tiPerd)
  Unit Delay1/1 -> DTC4/1
  DTC4/1 -> Add2/1
  DTC2/1 -> Add1/1
  DTC8/1 -> ISP_agRtrElecAtan2/1  "ISP_agRtrElecAtan2"
  exAtan2/1 -> DTC8/1, Add3/1, Unit Delay2/1
  Unit Delay2/1 -> Add3/2
  Add3/1 -> DTC6/1
  Gain/1 -> PT1/2
  Divide/1 -> Saturation/1
  PT1/1 -> ISP_frqElecCaln/1, Position PI Observer/1(frqCal)  "ISP_frqElecCaln"
  DTC6/1 -> Divide/1
  tiPerd1/1 -> Gain/1, Gain1/1
  Gain1/1 -> Divide/2
  kiRslvPI/1 -> Position PI Observer/4(Ki)
  kpRslvPI/1 -> Position PI Observer/5(Kp)
  Saturation/1 -> PT1/1
  sinH/1 -> Add4/1
  sinL/1 -> Add4/2
  Add4/1 -> DTC3/1
  Add5/1 -> DTC1/1
  cosH/1 -> Add5/1
  cosL/1 -> Add5/2

== system Monitor/ISP/ISP_Ana/ISP_AnaCalnUdcLnk ==
  note: 20180926
      | Change facAdc2uDclnkMon_C to 1 as the input monitor dclink voltage comes from CAN
  CddHvMcu_dataDclnkRaw : Inport
  DTC1 : DataTypeConversion  OutDataTypeStr=single  SaturateOnIntegerOverflow=off  RndMeth=Floor
  Divide : Product  Inputs=*/
  PT1 : MathLib/PT1
  Product3 : Product  OutDataTypeStr=single
  dtPT1UdcLink1 : Constant  Value=Tsw  OutDataTypeStr=single
  facAdc2uDclnk_C : Constant  Value=facAdc2uDclnkMon_C
      mask Display:
      | tmpx = get_param(gcbh,'Value');
      | a= evalin('base',[tmpx,'.Value;']);
      | disp([tmpx,': ',num2str(a)]);
  tauUdcPT1_C : Constant  Value=tauUdcPT1Mon_C
      mask Display:
      | tmpx = get_param(gcbh,'Value');
      | a= evalin('base',[tmpx,'.Value;']);
      | disp([tmpx,': ',num2str(a)]);
  ISP_uDcFltMon : Outport  VectorParamsAs1DForOutWhenUnconnected=off
  wires:
  Divide/1 -> PT1/2
  CddHvMcu_dataDclnkRaw/1 -> DTC1/1
  facAdc2uDclnk_C/1 -> Product3/2
  PT1/1 -> ISP_uDcFltMon/1  "ISP_uDcFltMon"
  Product3/1 -> PT1/1
  DTC1/1 -> Product3/1
  tauUdcPT1_C/1 -> Divide/2
  dtPT1UdcLink1/1 -> Divide/1

== system Monitor/ISP/ISP_Ana/ISP_AnaCalnUpha ==
  dataUPha : Inport
  Bus Creator : BusCreator  Inputs=3
  Bus Selector : BusSelector  OutputSignals=SAQ_DUTY1,SAQ_DUTY2,SAQ_DUTY3
  sub : Sum  Inputs=+++  OutDataTypeStr=single
  sub1 : Sum  Inputs=+-  OutDataTypeStr=single
  sub2 : Sum  Inputs=+-  OutDataTypeStr=single
  sub3 : Sum  Inputs=+-  OutDataTypeStr=single
  ISP_uPha : Outport  VectorParamsAs1DForOutWhenUnconnected=off
  wires:
  Bus Creator/1 -> ISP_uPha/1
  Bus Selector/1 -> sub/1, sub1/1  "<SAQ_DUTY1>"
  Bus Selector/2 -> sub/2, sub2/1  "<SAQ_DUTY2>"
  Bus Selector/3 -> sub3/1, sub/3  "<SAQ_DUTY3>"
  sub/1 -> sub3/2, sub2/2, sub1/2
  sub2/1 -> Bus Creator/2
  sub1/1 -> Bus Creator/1
  sub3/1 -> Bus Creator/3
  dataUPha/1 -> Bus Selector/1

== system Monitor/PMC/PMC_PsmMdl/MCT_GenSigCalcn ==
  ISP_Isd : Inport
  ISP_Isq : Inport  Port=2
  DTC2 : DataTypeConversion  OutDataTypeStr=single  SaturateOnIntegerOverflow=off  RndMeth=Floor
  DTC6 : DataTypeConversion  OutDataTypeStr=single  SaturateOnIntegerOverflow=off  RndMeth=Floor
  PT2 : MathLib/PT1
  PT3 : MathLib/PT1
  tauPT1Isd : Constant  Value=Tsw/0.001  OutDataTypeStr=single
  tauPT1Isq : Constant  Value=Tsw/0.001  OutDataTypeStr=single
  ISP_iDaFild : Outport  VectorParamsAs1DForOutWhenUnconnected=off
  ISP_iQaFild : Outport  Port=2  VectorParamsAs1DForOutWhenUnconnected=off
  wires:
  DTC2/1 -> ISP_iQaFild/1
  ISP_Isq/1 -> PT3/1
  tauPT1Isq/1 -> PT3/2
  DTC6/1 -> ISP_iDaFild/1
  ISP_Isd/1 -> PT2/1
  tauPT1Isd/1 -> PT2/2
  PT3/1 -> DTC2/1
  PT2/1 -> DTC6/1
